simulink model "SingleRigidBody"  (R2018a)
settings: Solver=ode3  StartTime=0.0  StopTime=Time  FixedStep=Ts  RelTol=1e-3  EnableMultiTasking=on
values from neighbouring files (symbols this model uses):
  ce1 = 0.053    [start.m]
  cp1 = 0.274    [start.m]
  ct1 = 0.048    [start.m]
  dot_q0 = [0 0 0]'    [start.m]
  g = 9.81    [start.m]
  I_e = 1.469    [start.m]
  I_t = 0.0319    [start.m]
  lcd = 0.10    (= 0.1)    [start.m]
  ldf = 0.17    [start.m]
  loc = 0.78    [start.m]
  m = (-mc*lob + mh *loc + mb*loa)/loc    (= 0.547587958974)    [start.m]
  mh = 1.8    [start.m]
  q0 = [0 0 0]'    [start.m]
  Ts = 0.005    [caldot_for_17.m]    (also in start.m)
libraries: dspsrcs4 x2
settings Model: Creator=chen  LastModifiedBy=yang
settings DataIOCC: LimitDataPoints=on  SaveFormat=Array  SignalLoggingSaveFormat=ModelDataLogs
settings OptimizationCC: LifeSpan=inf
settings DebuggingCC: SolverPrmCheckMsg=warning  MultiTaskDSMMsg=warning  MultiTaskCondExecSysMsg=none  SFUnexpectedBacktrackingDiag=warning  SFNoUnconditionalDefaultTransitionDiag=warning  SFExecutionAtInitializationDiag=none
settings HardwareCC: ProdBitPerPointer=32  ProdBitPerSizeT=32  ProdBitPerPtrDiffT=32  ProdLargestAtomicFloat=None  ProdIntDivRoundTo=Undefined  ProdEndianess=Unspecified  ProdWordSize=32  ProdHWDeviceType=32-bit Generic
settings ModelReferenceCC: PropagateSignalLabelsOutOfModel=off
settings CodeAppCC: StateflowObjectComments=on
settings GRTTargetCC: TargetLangStandard=C89/C90 (ANSI)  GeneratePreprocessorConditionals=Disable all
settings ConfigComp: CovMetricSettings=dw  CovHtmlReporting=on  CovSaveCumulativeToWorkspaceVar=on  CovSaveSingleToWorkspaceVar=on  CovExternalEMLEnable=off  CovSFcnEnable=off

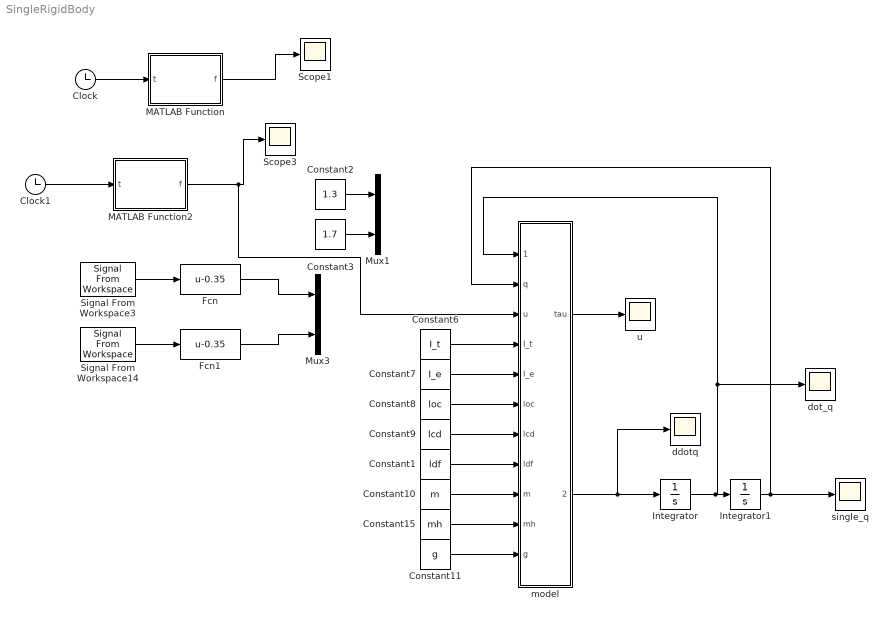
== system SingleRigidBody ==
  Clock : Clock
  Clock1 : Clock
  Constant1 : Constant  Value=ldf
  Constant10 : Constant  Value=m
  Constant11 : Constant  Value=g
  Constant15 : Constant  Value=mh
  Constant2 : Constant  Value=1.3
  Constant3 : Constant  Value=1.7
  Constant6 : Constant  Value=I_t
  Constant7 : Constant  Value=I_e
  Constant8 : Constant  Value=loc
  Constant9 : Constant  Value=lcd
  Fcn : Fcn  Expr=u-0.35
  Fcn1 : Fcn  Expr=u-0.35
  Integrator : Integrator  InitialCondition=dot_q0
  Integrator1 : Integrator  InitialCondition=q0
  MATLAB Function : MATLAB Function  TreatAsAtomicUnit=on
  MATLAB Function2 : MATLAB Function  TreatAsAtomicUnit=on
  Mux1 : Mux  Inputs=2
  Mux3 : Mux  Inputs=2
  Scope1 : Scope
  Scope3 : Scope
  Signal From Workspace14 : dspsrcs4/Signal From Workspace  X=F1  Ts=Ts  nsamps=1  OutputAfterFinalValue=Setting to zero  ignoreOrWarnInputAndFrameLengths=off  OutputFrames=on
  Signal From Workspace3 : dspsrcs4/Signal From Workspace  X=F2  Ts=Ts  nsamps=1  OutputAfterFinalValue=Setting to zero  ignoreOrWarnInputAndFrameLengths=off  OutputFrames=on
  ddotq : Scope
  dot_q : Scope
  model : MATLAB Function  TreatAsAtomicUnit=on
  single_q : Scope
  u : Scope
  wires:
  Integrator/1 -> dot_q/1, model/1(dot_q), Integrator1/1
  Constant6/1 -> model/4(I_t)
  Constant7/1 -> model/5(I_e)
  Constant8/1 -> model/6(loc)
  Constant9/1 -> model/7(lcd)
  Constant10/1 -> model/9(m)
  Constant11/1 -> model/11(g)
  Integrator1/1 -> model/2(q), single_q/1
  model/2(ddot_q) -> Integrator/1, ddotq/1
  Constant15/1 -> model/10(mh)
  model/1(tau) -> u/1
  Constant1/1 -> model/8(ldf)
  Clock/1 -> MATLAB Function/1(t)
  Clock1/1 -> MATLAB Function2/1(t)
  Signal From Workspace14/1 -> Fcn1/1
  Signal From Workspace3/1 -> Fcn/1
  Fcn/1 -> Mux3/1
  Fcn1/1 -> Mux3/2
  Constant2/1 -> Mux1/1
  Constant3/1 -> Mux1/2
  MATLAB Function/1(f) -> Scope1/1
  MATLAB Function2/1(f) -> model/3(u), Scope3/1

== matlab function SingleRigidBody/MATLAB Function2 ==
  data: t input; f output
function f = fcn(t)
f1 = 0;
f2 = 0;
if t>0&&t<25
    f1 = 1.7;
    f2 = 1.2;
elseif t>=25
    f1 = 1.3;
    f2 = 1.6;
end
f = [f1;f2];

== matlab function SingleRigidBody/MATLAB Function ==
  data: t input; f output
function f = fcn(t)
f1 = 0;
f2 = 0;
if t>=0&&t<30
    f1 = 1.5;
    f2 = 1.5;
elseif t>=30
    f1 = 1.7;
    f2 = 1.2;
end
f = [f1;f2];

== matlab function SingleRigidBody/model ==
  data: tau output; dot_q input; ddot_q output; q input; u input; I_t input; I_e input; loc input; lcd input; ldf input; m input; mh input; g input; cp1 parameter; ce1 parameter; ct1 parameter
function [tau,ddot_q] = fcn(dot_q,q,u,I_t,I_e,loc,lcd,ldf,m,mh,g, cp1, ce1, ct1)
I_psi = I_e;
dot_psai = dot_q(1);
dot_epsilon = dot_q(2);
dot_theta = dot_q(3);
psai = q(1);
epsilon = q(2);
theta = q(3);
M = [-I_t*sin(epsilon) 0 I_t;
     I_e*cos(epsilon)*sin(theta) I_e*cos(theta) 0;
     I_psi*cos(epsilon)*cos(theta) -I_psi*sin(theta) 0];
C = [(I_e-I_t)*cos(epsilon)*dot_epsilon -I_e*cos(epsilon)*dot_psai 0;
     (I_t-I_e)*sin(epsilon)*sin(theta)*dot_epsilon+(I_psi-I_t)*sin(epsilon)*cos(epsilon)*cos(theta)*dot_psai  -I_psi*sin(epsilon)*sin(theta)*dot_psai ...
     -I_t*sin(theta)*dot_epsilon+I_t*cos(epsilon)*cos(theta)*dot_psai;
     (I_t-I_psi)*sin(epsilon)*cos(theta)*dot_epsilon+(I_t-I_e)*cos(epsilon)*sin(epsilon)*sin(theta)*dot_psai -I_e*sin(epsilon)*cos(theta)*dot_psai ...
     -I_t*cos(theta)*dot_epsilon-I_t*cos(epsilon)*sin(theta)*dot_psai ]; 
% C = zeros(3,3);
% G = [-lcd*cos(epsilon)*sin(theta)*mh*g;
%      lcd*sin(epsilon)*mh*g-loc*cos(epsilon)*cos(theta)*m*g;
%      loc*cos(epsilon)*sin(theta)*m*g]; 
%  R =   [-cp1*I_psi 0 0;0 -ce1*I_e 0;0 0 -ct1*I_t];  %正负号疑惑
 R =   [cp1*I_psi 0 0;0 ce1*I_e 0;0 0 ct1*I_t];  %正负号疑惑
 G = [0;
     loc*cos(epsilon)*cos(theta)*m*g;
     -loc*cos(epsilon)*sin(theta)*m*g];   

tau = [ldf*(u(1) - u(2)); loc*(u(1) + u(2));0];
 ddot_q = ((tau - C*dot_q -R*dot_q  - G)\M)';
%ddot_q = inv(M)*(B*tau - C - G);
